simulink model "sysgenIIR_DFormI_Float"  (Simulink 7.5)
settings: Solver=VariableStepDiscrete  SolverMode=SingleTasking  StartTime=0.0  StopTime=20000  RelTol=1e-3
PreLoadFcn:
  | xlrequire('PreLoadFcn')
values from neighbouring files (symbols this model uses):
  Fs = 1 ./ block_data.params.XIncr    [sdspfscope2_r13.m]
undefined symbols (not defined in the file or in its folder): a1, a2, b0, b1, b2, One, sided
libraries: xbsIndex_r4 x59, dspobslib x6, dspstat3 x4, simulink x4, dspswit3 x2, dspsnks4 x2, xbsCopyrightNotice_r4 x1, dspsrcs4 x1
settings Model: Creator=alexc  LastModifiedBy=arvinds
settings DataIOCC: SignalLoggingName=sigsOut
settings OptimizationCC: BlockReduction=off  BooleanDataType=off  InlineInvariantSignals=on  InitFltsAndDblsToZero=on
settings DebuggingCC: SaveWithParameterizedLinksMsg=none  SignalResolutionControl=TryResolveAllWithWarning  SolverPrmCheckMsg=none  MultiTaskDSMMsg=warning  MultiTaskCondExecSysMsg=none  StrictBusMsg=None
settings HardwareCC: TargetUnknown=on
settings RTWCC: IncludeERTFirstTime=on
settings GRTTargetCC: TargetFcnLib=ansi_tfl_tmw.mat

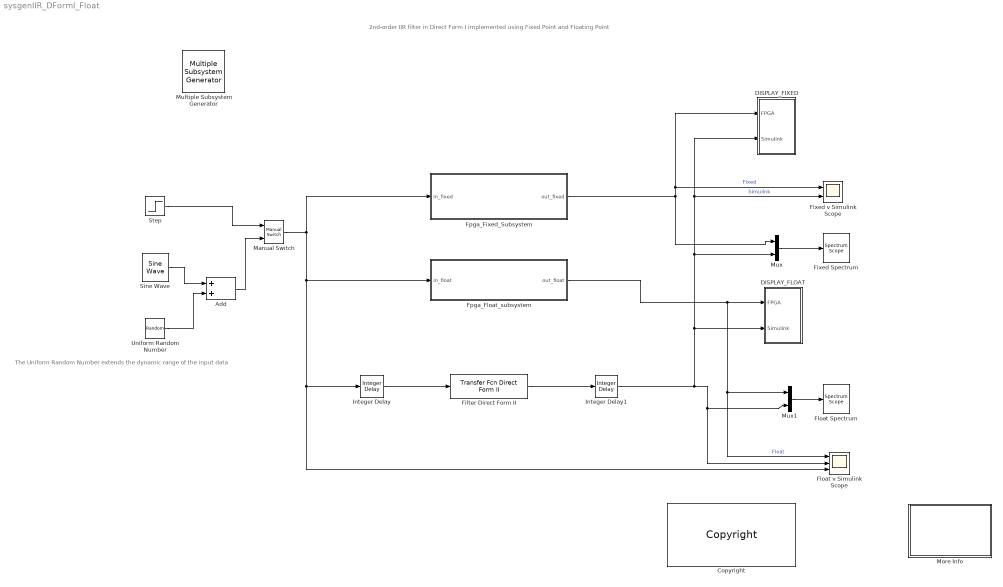
== system sysgenIIR_DFormI_Float ==
  note: 2nd-order IIR filter in Direct Form I
      | implemented using Fixed Point  and Floating Point
  note: The Uniform Random Number
      | extends the dynamic range of the input data
  Add : Sum
  Copyright : xbsCopyrightNotice_r4/Copyright  copyrighttext="Copyright (c) 2011  by  Xilinx, Inc. All rights reserved.<br><br>This file contains proprietary, confidential information of Xilinx, Inc., is distributed under license from Xilinx, Inc., and may be used, copied and/or disclosed only pursuant to the terms of a valid license agreement with Xilinx, Inc. Xilinx hereby grants you a license to use this file solely for design, simulation, implementation and creation of design files limited to Xilinx devices or technologies. Use with non-Xilinx devices or technologies is expressly prohibited and immediately terminates your license unless covered by a separate agreement.<br><br>Xilinx is providing this design, code, or information \"as-is\" solely for use in developing programs and solutions for Xilinx devices, with no obligation on the part of Xilinx to provide support. By providing this design, code, or information as one possible implementation of this feature, application or standard, Xilinx is making no representation that this implementation is free from any claims of infringement. You are responsible for obtaining any rights you may require for your implementation. Xilinx expressly disclaims any warranty whatsoever with respect to the adequacy of the implementation, including but not limited to any warranties or representations that this implementation is free from claims of infringement, implied warranties of merchantability or fitness for a particular purpose.<br><br>Xilinx products are not intended for use in life support appliances, devices, or systems. Use in such applications is expressly prohibited.<br><br>Any modifications that are made to the Source Code are done at the user's sole risk and will be unsupported.<br><br>This copyright and support notice must be retained as part of this text at all times. (c) Copyright 1995-2011 Xilinx, Inc. All rights reserved."  block_type=copyright
      settings: block_version=10.1.00
      settings: infoedit=|
      | Copyright(C) 2008 by  Xilinx, Inc. All rights reserved.<br>
      | <br>
      | This file contains proprietary, confidential information of Xilinx, Inc., is distributed under license
      | from Xilinx, Inc., and may be used, copied and/or disclosed only pursuant to the terms of a valid license
      | agreement with Xilinx, Inc. Xilinx hereby grants you a license to use this file solely for design,
      | simulation, implementation and creation of design files limited to Xilinx devices or technologies. Use
      | with non-Xilinx devices or technologies is expressly prohibited and immediately terminates your license
      | unless covered by a separate agreement.<br>
      | <br>
      | Xilinx is providing this design, code, or information "as-is" solely for use in developing programs and
      | solutions for Xilinx devices, with no obligation on the part of Xilinx to provide support. By providing
      | this design, code, or information as one possible implementation of this feature, application or standard,
      | Xilinx is making no representation that this implementation is free from any claims of infringement. You
      | are responsible for obtaining any rights you may require for your implementation. Xilinx expressly disclaims
      | any warranty whatsoever with respect to the adequacy of the implementation, including but not limited to any
      | warranties or representations that this implementation is free from claims of infringement, implied warranties
      | of merchantability or fitness for a particular purpose.<br>
      | <br>
      | Xilinx products are not intended for use in life support appliances, devices, or systems. Use in such
      | applications is expressly prohibited.<br>
      | <br>
      | Any modifications that are made to the Source Code are done at the user's sole risk and will be unsupported.<br>
      | <br>
      | This copyright and support notice must be retained as part of this text at all times.
      | (c) Copyright 1995-2008 Xilinx, Inc. All rights reserved.
  DISPLAY_FIXED : Subsystem  TreatAsAtomicUnit=on
  DISPLAY_FLOAT : Subsystem  TreatAsAtomicUnit=on
  Filter Direct Form II : simulink/Additional Math & Discrete/Additional Discrete/Transfer Fcn Direct Form II  SystemSampleTime=-1  NumCoefVec=[1 -1.6929 1]  DenCoefVec=[1.2591 0.82538]  vinit=0.0  DoSatur=off
  Fixed Spectrum : dspsnks4/Spectrum Scope  DialogController=dspdialog.SpectrumScope  DialogControllerArgs=DataTag8  SystemSampleTime=-1  ScopeProperties=off  Domain=Frequency  HorizSpan=1  UseBuffer=on  BufferSize=512  Overlap=0  inpFftLenInherit=off  FFTlength=128  numAvg=1  DisplayProperties=off  AxisGrid=on  Memory=off  FrameNumber=on  AxisLegend=on  AxisZoom=off  OpenScopeAtSimStart=on  OpenScopeImmediately=off  FigPos=[1105 390 423 236]  AxisProperties=off  XUnits=Hertz  XRange=One-sided ([0...Fs/2])  XDisplay=0  InheritXIncr=off  XIncr=1/50e6  XLabel=Samples  XLimit=Auto  YUnits=dBW/Hertz  XMax=1  XMin=0  YLabel=Magnitude, dB  LineProperties=off  LineColors=[0 1 1]|[0 0 1]|[0.1 0.6 0.1]  wintypeSpecScope=Hann  RsSpecScope=50  betaSpecScope=5  winsampSpecScope=Periodic  XAxisParamsVer=6.9
      settings: YMin=-100  YMax=0
  Fixed v Simulink Scope : Scope  NumInputPorts=2
      settings: YMin=-150~-125  YMax=150~125
  Float Spectrum : dspsnks4/Spectrum Scope  DialogController=dspdialog.SpectrumScope  DialogControllerArgs=DataTag9  SystemSampleTime=-1  ScopeProperties=off  Domain=Frequency  HorizSpan=1  UseBuffer=on  BufferSize=512  Overlap=0  inpFftLenInherit=off  FFTlength=128  numAvg=1  DisplayProperties=off  AxisGrid=on  Memory=off  FrameNumber=on  AxisLegend=on  AxisZoom=off  OpenScopeAtSimStart=on  OpenScopeImmediately=off  FigPos=[1105 390 423 236]  AxisProperties=off  XUnits=Hertz  XRange=One-sided ([0...Fs/2])  XDisplay=0  InheritXIncr=off  XIncr=1/50e6  XLabel=Samples  XLimit=Auto  YUnits=dBW/Hertz  XMax=1  XMin=0  YLabel=Magnitude, dB  LineProperties=off  LineColors=[0 1 1]|[0 0 1]|[0.1 0.6 0.1]  wintypeSpecScope=Hann  RsSpecScope=50  betaSpecScope=5  winsampSpecScope=Periodic  XAxisParamsVer=6.9
      settings: YMin=-100  YMax=0
  Float v Simulink Scope : Scope  NumInputPorts=3
      settings: YMin=-100~-100~-20  YMax=100~100~20
  Fpga_Fixed_Subsystem : Subsystem
  Fpga_Float_subsystem : Subsystem
  Integer Delay : simulink/Discrete/Integer Delay  vinit=0.0  samptime=1/Fs  NumDelays=5
  Integer Delay1 : simulink/Discrete/Integer Delay  vinit=0.0  samptime=1/Fs  NumDelays=2
  Manual Switch : simulink/Signal Routing/Manual Switch  SystemSampleTime=-1  sw=0  action=0  varsize=off
  More Info : Subsystem
      mask Display: disp('Double click\n for\n more information.')
  Multiple Subsystem Generator : xbsIndex_r4/Multiple Subsystem Generator  Tag=xlStitcher  block_type=multiple_subsystem_generator
      settings: infoedit=Multiple Subsystem\nGenerator  block_version=13.3
  Mux : Mux  Inputs=2
  Mux1 : Mux  Inputs=2
  Sine Wave : dspsrcs4/Sine Wave  Amplitude=9.99  Frequency=Fs/10  Phase=0  SampleMode=Discrete  OutComplex=Real  CompMethod=Trigonometric fcn  TableSize=Speed  SampleTime=1/Fs  SamplesPerFrame=1  dataType=double  wordLen=16  udDataType=sfix(16)  fracBitsMode=Best precision  numFracBits=14  ResetState=Restart at time zero
  Step : Step  Before=1  After=0  SampleTime=1/Fs
  Uniform Random Number : UniformRandomNumber  Minimum=-7  Maximum=7  SampleTime=1/Fs
  wires:
  Filter Direct Form II/1 -> Integer Delay1/1
  Fpga_Fixed_Subsystem/1(out_fixed) -> Mux/1, DISPLAY_FIXED/1(FPGA), Fixed v Simulink Scope/1  "Fixed"
  Step/1 -> Manual Switch/1
  Manual Switch/1 -> Fpga_Fixed_Subsystem/1(in_fixed), Fpga_Float_subsystem/1(in_float), Float v Simulink Scope/3, Integer Delay/1
  Integer Delay1/1 -> DISPLAY_FLOAT/2(Simulink), Mux/2, DISPLAY_FIXED/2(Simulink), Fixed v Simulink Scope/2, Mux1/2, Float v Simulink Scope/2  "Simulink"
  Mux/1 -> Fixed Spectrum/1
  Fpga_Float_subsystem/1(out_float) -> DISPLAY_FLOAT/1(FPGA), Mux1/1, Float v Simulink Scope/1  "Float"
  Mux1/1 -> Float Spectrum/1
  Uniform Random Number/1 -> Add/2
  Sine Wave/1 -> Add/1
  Add/1 -> Manual Switch/2
  Integer Delay/1 -> Filter Direct Form II/1

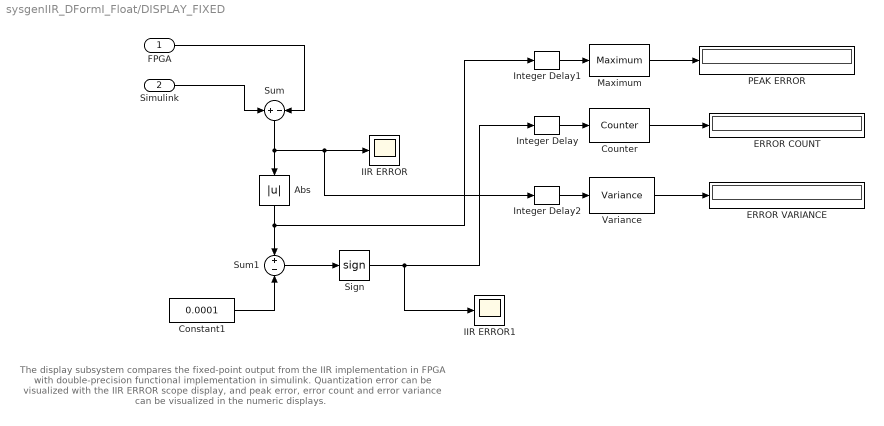
== system sysgenIIR_DFormI_Float/DISPLAY_FIXED ==
  note: The display subsystem compares the fixed-point output from the IIR implementation in FPGA
      | with double-precision functional implementation in simulink. Quantization error can be visualized
      | with the IIR ERROR scope display, and peak error, error count and error variance can be visualized
      | in the numeric displays.
  FPGA : Inport
  Simulink : Inport  Port=2
  Abs : Abs  SaturateOnIntegerOverflow=on
  Constant1 : Constant  Value=0.0001
  Counter : dspswit3/Counter  Direction=Up  CountEvent=Non-zero sample  CounterSize=User defined  MaxCount=200000000  InitialCount=0  Output=Count  HitValue=32  ResetInput=off  SamplesPerFrame=1  Ts=1  CntDtype=double  HitDtype=Logical
  ERROR COUNT : Display
  ERROR VARIANCE : Display
      settings: Format=long_e
  IIR ERROR : Scope
      settings: TimeRange=10000  YMin=-0.0006  YMax=0.0005  SaveName=ScopeData2
  IIR ERROR1 : Scope
      settings: TimeRange=10000  YMin=-0.0006  YMax=0.0005  SaveName=ScopeData3
  Integer Delay : dspobslib/Integer Delay  delay=1  ic=0  reset_popup=None
  Integer Delay1 : dspobslib/Integer Delay  delay=1  ic=0  reset_popup=None
  Integer Delay2 : dspobslib/Integer Delay  delay=1  ic=0  reset_popup=None
  Maximum : dspstat3/Maximum  DialogController=dspDDGCreate  DialogControllerArgs=DataTag1  fcn=Running  reset=None  indexBase=One  operateOver=Each column  Dimension=1  colComp=on  operation=maximum  roiEnable=off  roiType=Rectangles  roiPortion=Entire ROI  roiOutput=Individual statistics for each ROI  roiFlag=off  accumDataTypeStr=Inherit: Same as product output  accumLastDataTypeStr=Inherit: Same as product output  roundingMode=Floor  overflowMode=off
  PEAK ERROR : Display
      settings: Format=long_e
  Sign : Signum
  Sum : Sum  Inputs=+-  SaturateOnIntegerOverflow=on  InputSameDT=on  OutDataTypeStr=Inherit: Same as first input
  Sum1 : Sum  Inputs=+-  SaturateOnIntegerOverflow=on  InputSameDT=on  OutDataTypeStr=Inherit: Same as first input
  Variance : dspstat3/Variance  DialogController=dspDDGCreate  DialogControllerArgs=DataTag3  run=on  reset_popup=None  directionMode=Each column  dimension=1  treatSBRowAsCol=on  roiEnable=off  roiType=Rectangles  roiPortion=Entire ROI  roiOutput=Individual statistics for each ROI  roiFlag=off  roundingMode=Floor  overflowMode=off
  wires:
  FPGA/1 -> Sum/2
  Simulink/1 -> Sum/1
  Sum/1 -> Abs/1, IIR ERROR/1, Integer Delay2/1
  Constant1/1 -> Sum1/2
  Abs/1 -> Sum1/1, Integer Delay1/1
  Sum1/1 -> Sign/1
  Sign/1 -> Integer Delay/1, IIR ERROR1/1
  Counter/1 -> ERROR COUNT/1
  Variance/1 -> ERROR VARIANCE/1
  Maximum/1 -> PEAK ERROR/1
  Integer Delay/1 -> Counter/1
  Integer Delay1/1 -> Maximum/1
  Integer Delay2/1 -> Variance/1

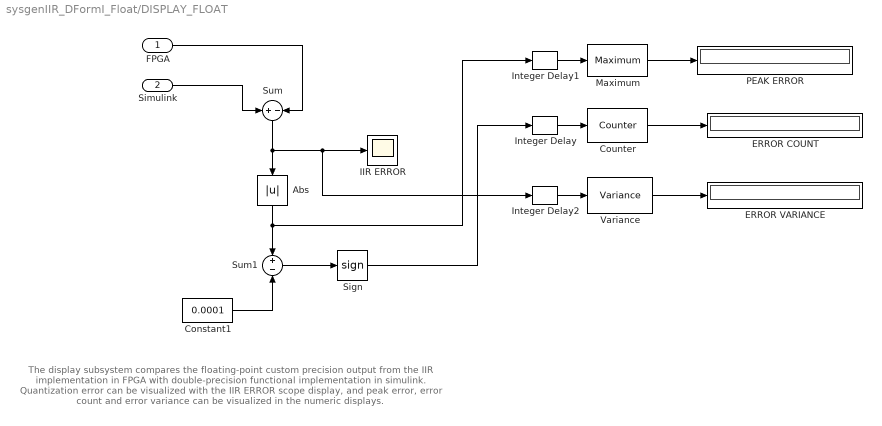
== system sysgenIIR_DFormI_Float/DISPLAY_FLOAT ==
  note: The display subsystem compares the floating-point custom precision output from the IIR implementation in FPGA
      | with double-precision functional implementation in simulink. Quantization error can be visualized
      | with the IIR ERROR scope display, and peak error, error count and error variance can be visualized
      | in the numeric displays.
  FPGA : Inport
  Simulink : Inport  Port=2
  Abs : Abs  SaturateOnIntegerOverflow=on
  Constant1 : Constant  Value=0.0001
  Counter : dspswit3/Counter  Direction=Up  CountEvent=Rising edge  CounterSize=User defined  MaxCount=200000000  InitialCount=0  Output=Count  HitValue=32  ResetInput=off  SamplesPerFrame=1  Ts=1  CntDtype=double  HitDtype=Logical
  ERROR COUNT : Display
  ERROR VARIANCE : Display
      settings: Format=long_e
  IIR ERROR : Scope
      settings: TimeRange=10000  YMin=-0.0006  YMax=0.0005  SaveName=ScopeData2
  Integer Delay : dspobslib/Integer Delay  delay=1  ic=0  reset_popup=None
  Integer Delay1 : dspobslib/Integer Delay  delay=1  ic=0  reset_popup=None
  Integer Delay2 : dspobslib/Integer Delay  delay=1  ic=0  reset_popup=None
  Maximum : dspstat3/Maximum  DialogController=dspDDGCreate  DialogControllerArgs=DataTag5  fcn=Running  reset=None  indexBase=One  operateOver=Each column  Dimension=1  colComp=on  operation=maximum  roiEnable=off  roiType=Rectangles  roiPortion=Entire ROI  roiOutput=Individual statistics for each ROI  roiFlag=off  accumDataTypeStr=Inherit: Same as product output  accumLastDataTypeStr=Inherit: Same as product output  roundingMode=Floor  overflowMode=off
  PEAK ERROR : Display
      settings: Format=long_e
  Sign : Signum
  Sum : Sum  Inputs=+-  SaturateOnIntegerOverflow=on  InputSameDT=on  OutDataTypeStr=Inherit: Same as first input
  Sum1 : Sum  Inputs=+-  SaturateOnIntegerOverflow=on  InputSameDT=on  OutDataTypeStr=Inherit: Same as first input
  Variance : dspstat3/Variance  DialogController=dspDDGCreate  DialogControllerArgs=DataTag7  run=on  reset_popup=None  directionMode=Each column  dimension=1  treatSBRowAsCol=on  roiEnable=off  roiType=Rectangles  roiPortion=Entire ROI  roiOutput=Individual statistics for each ROI  roiFlag=off  roundingMode=Floor  overflowMode=off
  wires:
  FPGA/1 -> Sum/2
  Simulink/1 -> Sum/1
  Sum/1 -> Abs/1, IIR ERROR/1, Integer Delay2/1
  Constant1/1 -> Sum1/2
  Abs/1 -> Sum1/1, Integer Delay1/1
  Sum1/1 -> Sign/1
  Sign/1 -> Integer Delay/1
  Counter/1 -> ERROR COUNT/1
  Variance/1 -> ERROR VARIANCE/1
  Maximum/1 -> PEAK ERROR/1
  Integer Delay/1 -> Counter/1
  Integer Delay1/1 -> Maximum/1
  Integer Delay2/1 -> Variance/1

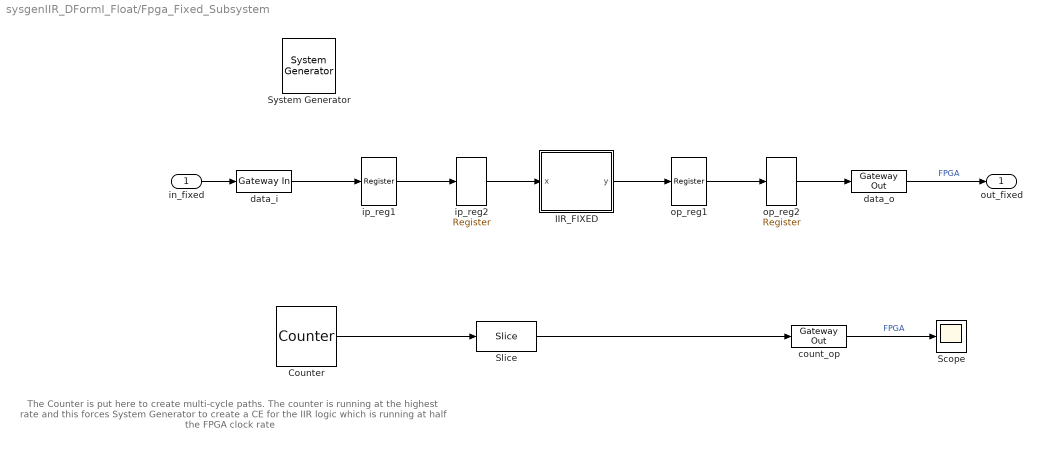
== system sysgenIIR_DFormI_Float/Fpga_Fixed_Subsystem ==
  note: The Counter is put here to create multi-cycle paths. The counter is running at the highest rate
      | and this forces System Generator  to create a CE for the IIR logic which is running at half the
      | FPGA clock rate
  in_fixed : Inport
  " System Generator" : xbsIndex_r4/ System Generator  Tag=genX  SystemSampleTime=-1  xilinxfamily=virtex6  part=xc6vlx240t  speed=-1  package=ff1156  synthesis_tool=XST  clock_wrapper=Clock Enables  directory=./fixed_timing  proj_type=Project Navigator  Synth_file=XST Defaults  Impl_file=ISE Defaults  testbench=off  simulink_period=1/(2*Fs)  sysclk_period=20  dcm_input_clock_period=100  incr_netlist=off  trim_vbits=According to Block Masks  dbl_ovrd=According to Block Masks  core_generation=According to Block Masks  run_coregen=off  deprecated_control=off  eval_field=0  block_type=sysgen
      settings: block_version=9.2.00
  Counter : xbsIndex_r4/Counter  cnt_type=Free Running  cnt_to=Inf  operation=Up  start_count=0  cnt_by_val=1  arith_type=Unsigned  n_bits=8  bin_pt=0  load_pin=off  rst=off  en=off  explicit_period=on  period=1/(2*Fs)  dbl_ovrd=off  use_behavioral_HDL=off  implementation=Fabric  block_type=counter
      settings: block_version=13.3
  IIR_FIXED : Subsystem
  Scope : Scope
      settings: SaveName=ScopeData5
  Slice : xbsIndex_r4/Slice  nbits=1  boolean_output=on  mode=Upper Bit Location + Width  bit1=0  base1=MSB of Input  bit0=0  base0=LSB of Input  dbl_ovrd=off  block_type=slice
      settings: block_version=13.3
  count_op : xbsIndex_r4/Gateway Out  hdl_port=off  timing_constraint=None  locs_specified=off  LOCs={}  block_type=gatewayout
      settings: infoedit="Gateway out block.  Converts Xilinx fixed point or floating-point type inputs into ouputs of type Simulink integer, double, or fixed point.<br><br>Hardware notes:  In hardware these blocks become top level output ports or are discarded, depending on how they are configured."  xl_area=[0 0 0 0 12 0 0]  block_version=VER_STRING_GOES_HERE
  data_i : xbsIndex_r4/Gateway In  gui_display_data_type=Fixed-point  arith_type="Signed  (2's comp)"  n_bits=data_width  bin_pt=data_binary_pt  preci_type=Single  exp_width=8  frac_width=24  quantization="Round  (unbiased: +/- Inf)"  overflow=Saturate  period=1/Fs  dbl_ovrd=off  timing_constraint=None  locs_specified=off  LOCs={}  hdl_port=on  block_type=gatewayin
      settings: infoedit="Gateway in block.  Converts inputs of type Simulink integer, double and fixed point to  Xilinx fixed point or floating-point data type.<br><br>Hardware notes:  In hardware these blocks become top level input ports."  xl_area=[0 0 0 0 12 0 0]  block_version=VER_STRING_GOES_HERE
  data_o : xbsIndex_r4/Gateway Out  hdl_port=on  timing_constraint=None  locs_specified=off  LOCs={}  block_type=gatewayout
      settings: infoedit="Gateway out block.  Converts Xilinx fixed point inputs into ouputs of type Simulink integer, double, or fixed point.<P><P>Hardware notes:  In hardware these blocks become top level output ports or are discarded, depending on how they are configured."  xl_area=[0 0 0 0 12 0 0]  block_version=VER_STRING_GOES_HERE
  ip_reg1 : xbsIndex_r4/Register  init=0  rst=off  en=off  dbl_ovrd=off  block_type=register
      settings: block_version=VER_STRING_GOES_HERE
  ip_reg2 : xbsIndex_r4/Register  init=0  rst=off  en=off  dbl_ovrd=off  block_type=register
      settings: block_version=VER_STRING_GOES_HERE
  op_reg1 : xbsIndex_r4/Register  init=0  rst=off  en=off  dbl_ovrd=off  block_type=register
      settings: block_version=VER_STRING_GOES_HERE
  op_reg2 : xbsIndex_r4/Register  init=0  rst=off  en=off  dbl_ovrd=off  block_type=register
      settings: block_version=VER_STRING_GOES_HERE
  out_fixed : Outport
  wires:
  data_i/1 -> ip_reg1/1
  ip_reg1/1 -> ip_reg2/1
  ip_reg2/1 -> IIR_FIXED/1(x)
  op_reg1/1 -> op_reg2/1
  IIR_FIXED/1(y) -> op_reg1/1
  op_reg2/1 -> data_o/1
  in_fixed/1 -> data_i/1
  data_o/1 -> out_fixed/1  "FPGA"
  count_op/1 -> Scope/1  "FPGA"
  Counter/1 -> Slice/1
  Slice/1 -> count_op/1

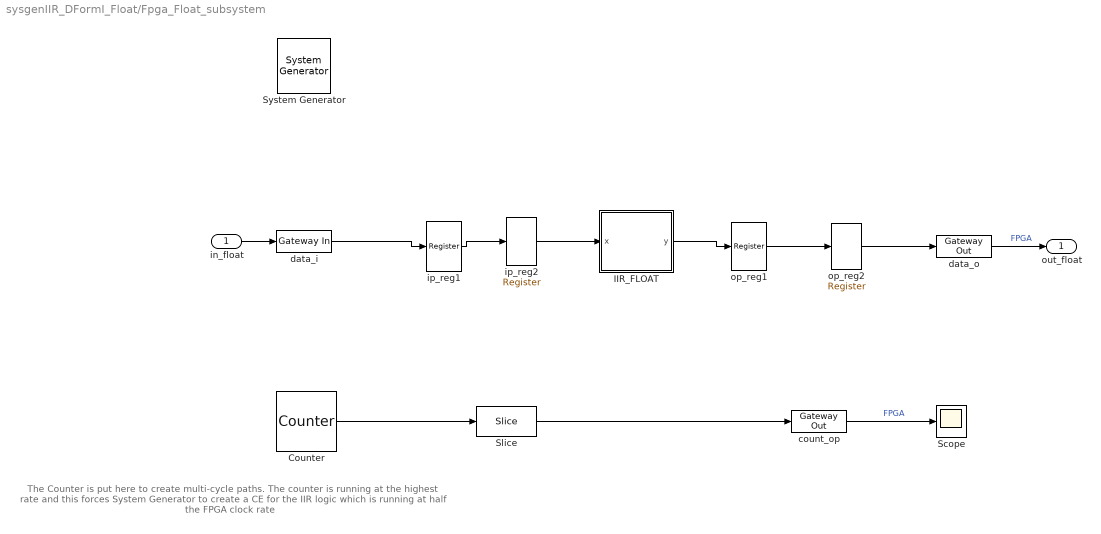
== system sysgenIIR_DFormI_Float/Fpga_Float_subsystem ==
  note: The Counter is put here to create multi-cycle paths. The counter is running at the highest rate
      | and this forces System Generator  to create a CE for the IIR logic which is running at half the
      | FPGA clock rate
  in_float : Inport
  " System Generator" : xbsIndex_r4/ System Generator  Tag=genX  SystemSampleTime=-1  xilinxfamily=virtex6  part=xc6vlx240t  speed=-1  package=ff1156  synthesis_tool=XST  clock_wrapper=Clock Enables  directory=./netlist  proj_type=Project Navigator  Synth_file=XST Defaults  Impl_file=ISE Defaults  testbench=off  simulink_period=1/(2*Fs)  sysclk_period=20  dcm_input_clock_period=100  incr_netlist=off  trim_vbits=According to Block Masks  dbl_ovrd=According to Block Masks  core_generation=According to Block Masks  run_coregen=off  deprecated_control=off  eval_field=0  block_type=sysgen
      settings: block_version=9.2.00
  Counter : xbsIndex_r4/Counter  cnt_type=Free Running  cnt_to=Inf  operation=Up  start_count=0  cnt_by_val=1  arith_type=Unsigned  n_bits=8  bin_pt=0  load_pin=off  rst=off  en=off  explicit_period=on  period=1/(2*Fs)  dbl_ovrd=off  use_behavioral_HDL=off  implementation=Fabric  block_type=counter
      settings: block_version=13.3
  IIR_FLOAT : Subsystem
  Scope : Scope
      settings: SaveName=ScopeData4
  Slice : xbsIndex_r4/Slice  nbits=1  boolean_output=on  mode=Upper Bit Location + Width  bit1=0  base1=MSB of Input  bit0=0  base0=LSB of Input  dbl_ovrd=off  block_type=slice
      settings: block_version=13.3
  count_op : xbsIndex_r4/Gateway Out  hdl_port=off  timing_constraint=None  locs_specified=off  LOCs={}  block_type=gatewayout
      settings: infoedit="Gateway out block.  Converts Xilinx fixed point or floating-point type inputs into ouputs of type Simulink integer, double, or fixed point.<br><br>Hardware notes:  In hardware these blocks become top level output ports or are discarded, depending on how they are configured."  xl_area=[0 0 0 0 12 0 0]  block_version=VER_STRING_GOES_HERE
  data_i : xbsIndex_r4/Gateway In  gui_display_data_type=Floating-point  arith_type=Floating-point  n_bits=data_width  bin_pt=data_binary_pt  preci_type=Custom  exp_width=fp_exp  frac_width=fp_frac  quantization="Round  (unbiased: +/- Inf)"  overflow=Saturate  period=1/Fs  dbl_ovrd=off  timing_constraint=None  locs_specified=off  LOCs={}  hdl_port=on  block_type=gatewayin
      settings: infoedit="Gateway in block.  Converts inputs of type Simulink integer, double and fixed point to  Xilinx fixed point or floating-point data type.<br><br>Hardware notes:  In hardware these blocks become top level input ports."  xl_area=[0 0 0 0 12 0 0]  block_version=VER_STRING_GOES_HERE
  data_o : xbsIndex_r4/Gateway Out  hdl_port=on  timing_constraint=None  locs_specified=off  LOCs={}  block_type=gatewayout
      settings: infoedit="Gateway out block.  Converts Xilinx fixed point inputs into ouputs of type Simulink integer, double, or fixed point.<P><P>Hardware notes:  In hardware these blocks become top level output ports or are discarded, depending on how they are configured."  xl_area=[0 0 0 0 12 0 0]  block_version=VER_STRING_GOES_HERE
  ip_reg1 : xbsIndex_r4/Register  init=0  rst=off  en=off  dbl_ovrd=off  block_type=register
      settings: block_version=VER_STRING_GOES_HERE
  ip_reg2 : xbsIndex_r4/Register  init=0  rst=off  en=off  dbl_ovrd=off  block_type=register
      settings: block_version=VER_STRING_GOES_HERE
  op_reg1 : xbsIndex_r4/Register  init=0  rst=off  en=off  dbl_ovrd=off  block_type=register
      settings: block_version=VER_STRING_GOES_HERE
  op_reg2 : xbsIndex_r4/Register  init=0  rst=off  en=off  dbl_ovrd=off  block_type=register
      settings: block_version=VER_STRING_GOES_HERE
  out_float : Outport
  wires:
  data_i/1 -> ip_reg1/1
  ip_reg1/1 -> ip_reg2/1
  ip_reg2/1 -> IIR_FLOAT/1(x)
  op_reg1/1 -> op_reg2/1
  IIR_FLOAT/1(y) -> op_reg1/1
  op_reg2/1 -> data_o/1
  in_float/1 -> data_i/1
  data_o/1 -> out_float/1  "FPGA"
  count_op/1 -> Scope/1  "FPGA"
  Counter/1 -> Slice/1
  Slice/1 -> count_op/1

== system sysgenIIR_DFormI_Float/More Info ==
  note: This design example shows two distinct FPGA implementations of a 2nd order IIR filter in Direct Form I,
      | and compares them to the double precision Simulink IIR filter block.
      |
      | The FPGA_FIXED_SUBSYSTEM is an IIR block 'IIIR_FIXED which is implemented with data input set to Fix32_27;
      | coefficients use 32 bit with 30 bits fractional and the adder tree usesFix32_24 notation
      |
      | The FPGA_FLOAT_SUBSYSTEM is an IIR block 'IIIR_FLOAT which is implemented using floating point block with custom
      | precision with exponent set to 7 bits and the fractional set to 20 bits
      | Therefore data and coefficients use Float_7_20
      |
      | Multiple display blocks allow the user to visualize the Power Spectrum  Density (PSD) of each
      | implementation as well as the quantization error in the DISPLAY block.
      |
      | The input is a sine wave with random noise added. if the random noise is small the fixed implementation gives good results
      | but as the dynamic range is increased the floating point implementation is better and when compared with an error window
      | the fixed implemenation is alway outside the error window.
      |
      | All the variables such as data width, coefficient width, Sample period, and coefficient values are
      | initialized in the sysgenIIR_DFormI_Float_PreLoadFcn.m file.
      |
      | A counter has been added here to create multi-cycle paths. The counter is running at the highest rate
      | and this forces System Generator  to create a CE for the IIR logic which is running at half the
      | FPGA clock rate
  note: 2nd-order IIR filter in Direct Form I
      | implemented using Fixed Point  and Floating Point

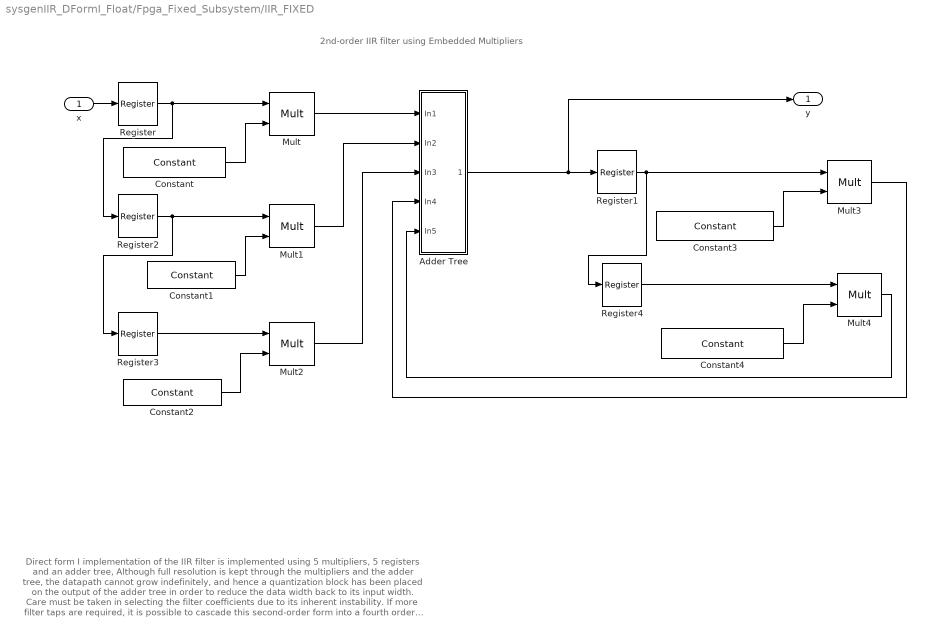
== system sysgenIIR_DFormI_Float/Fpga_Fixed_Subsystem/IIR_FIXED ==
  note: Direct form I implementation of the IIR filter is implemented using 5 multipliers, 5 registers
      | and an adder tree, Although full resolution is kept through the multipliers and the
      | adder tree, the datapath cannot grow indefinitely, and hence a quantization block has
      | been placed on the output of the adder tree in order to reduce the data width back to its
      | input width.
      | Care must be taken in selecting the filter coefficients due to its inherent instability.
      |
      | If more filter taps are required, it is possible to cascade this second-order form into a
      | fourth order cascaded filter, combine them in parallel or time share the current design
      | by saving multiple sets of coefficients in distributed memories. Similarly, the time sharing
      | approach can be used for multi-channel requirements, in which case, the coefficients can
      | be saved in distributed memories or block memories depending on the number of channels.
      |
      | Because of the feedback loop, no latency and hence no pipelining is possible in this design.
      | It is for this reason, fairly difficult to achieve high sample rate with such implementation.
  note: 2nd-order IIR filter using Embedded Multipliers
  x : Inport
  Adder Tree : Subsystem
  Constant : xbsIndex_r4/Constant  const=b0  gui_display_data_type=Fixed-point  arith_type=Signed (2's comp)  n_bits=coef_width  bin_pt=coef_binary_pt  preci_type=Single  exp_width=8  frac_width=24  explicit_period=off  period=1  equ=P=C  opselect=C  inp2=PCIN>>17  opr=+  inp1=P  carry=CIN  dbl_ovrd=off  block_type=constant
      settings: block_version=VER_STRING_GOES_HERE
  Constant1 : xbsIndex_r4/Constant  const=b1  gui_display_data_type=Fixed-point  arith_type=Signed (2's comp)  n_bits=coef_width  bin_pt=coef_binary_pt  preci_type=Single  exp_width=8  frac_width=24  explicit_period=off  period=1  equ=P=C  opselect=C  inp2=PCIN>>17  opr=+  inp1=P  carry=CIN  dbl_ovrd=off  block_type=constant
      settings: block_version=VER_STRING_GOES_HERE
  Constant2 : xbsIndex_r4/Constant  const=b2  gui_display_data_type=Fixed-point  arith_type=Signed (2's comp)  n_bits=coef_width  bin_pt=coef_binary_pt  preci_type=Single  exp_width=8  frac_width=24  explicit_period=off  period=1  equ=P=C  opselect=C  inp2=PCIN>>17  opr=+  inp1=P  carry=CIN  dbl_ovrd=off  block_type=constant
      settings: block_version=VER_STRING_GOES_HERE
  Constant3 : xbsIndex_r4/Constant  const=-a1  gui_display_data_type=Fixed-point  arith_type=Signed (2's comp)  n_bits=coef_width  bin_pt=coef_binary_pt  preci_type=Single  exp_width=8  frac_width=24  explicit_period=off  period=1  equ=P=C  opselect=C  inp2=PCIN>>17  opr=+  inp1=P  carry=CIN  dbl_ovrd=off  block_type=constant
      settings: block_version=VER_STRING_GOES_HERE
  Constant4 : xbsIndex_r4/Constant  const=-a2  gui_display_data_type=Fixed-point  arith_type=Signed (2's comp)  n_bits=coef_width  bin_pt=coef_binary_pt  preci_type=Single  exp_width=8  frac_width=24  explicit_period=off  period=1  equ=P=C  opselect=C  inp2=PCIN>>17  opr=+  inp1=P  carry=CIN  dbl_ovrd=off  block_type=constant
      settings: block_version=VER_STRING_GOES_HERE
  Mult : xbsIndex_r4/Mult  precision=User Defined  arith_type="Signed  (2's comp)"  n_bits=32  bin_pt=24  quantization="Round  (unbiased: +/- Inf)"  overflow=Saturate  en=off  latency=1  dbl_ovrd=off  use_behavioral_HDL=off  opt=Speed  use_embedded=on  optimum_pipeline=off  pipeline=off  use_rpm=off  placement_style=Rectangular shape  block_type=mult
      settings: xl_area=[0 0 0 0 0 1 0]  block_version=VER_STRING_GOES_HERE
  Mult1 : xbsIndex_r4/Mult  precision=User Defined  arith_type="Signed  (2's comp)"  n_bits=32  bin_pt=24  quantization="Round  (unbiased: +/- Inf)"  overflow=Saturate  en=off  latency=1  dbl_ovrd=off  use_behavioral_HDL=off  opt=Speed  use_embedded=on  optimum_pipeline=off  pipeline=off  use_rpm=off  placement_style=Rectangular shape  block_type=mult
      settings: xl_area=[0 0 0 0 0 1 0]  block_version=VER_STRING_GOES_HERE
  Mult2 : xbsIndex_r4/Mult  precision=User Defined  arith_type="Signed  (2's comp)"  n_bits=32  bin_pt=24  quantization="Round  (unbiased: +/- Inf)"  overflow=Saturate  en=off  latency=1  dbl_ovrd=off  use_behavioral_HDL=off  opt=Speed  use_embedded=on  optimum_pipeline=off  pipeline=off  use_rpm=off  placement_style=Rectangular shape  block_type=mult
      settings: xl_area=[0 0 0 0 0 1 0]  block_version=VER_STRING_GOES_HERE
  Mult3 : xbsIndex_r4/Mult  precision=User Defined  arith_type="Signed  (2's comp)"  n_bits=32  bin_pt=24  quantization=Truncate  overflow=Wrap  en=off  latency=0  dbl_ovrd=off  use_behavioral_HDL=off  opt=Speed  use_embedded=on  optimum_pipeline=off  pipeline=off  use_rpm=off  placement_style=Rectangular shape  block_type=mult
      settings: xl_area=[0 0 0 0 0 1 0]  block_version=VER_STRING_GOES_HERE
  Mult4 : xbsIndex_r4/Mult  precision=User Defined  arith_type="Signed  (2's comp)"  n_bits=32  bin_pt=24  quantization=Truncate  overflow=Wrap  en=off  latency=0  dbl_ovrd=off  use_behavioral_HDL=off  opt=Speed  use_embedded=on  optimum_pipeline=off  pipeline=off  use_rpm=off  placement_style=Rectangular shape  block_type=mult
      settings: xl_area=[0 0 0 0 0 1 0]  block_version=VER_STRING_GOES_HERE
  Register{,1..4} (5 alike) : xbsIndex_r4/Register  init=0  rst=off  en=off  dbl_ovrd=off  block_type=register
      settings: xl_area=[6 12 0 0 0 0 0]  block_version=VER_STRING_GOES_HERE
  y : Outport
  wires:
  x/1 -> Register/1
  Register1/1 -> Mult3/1, Register4/1
  Constant3/1 -> Mult3/2
  Mult4/1 -> Adder Tree/5(In5)
  Mult3/1 -> Adder Tree/4(In4)
  Constant4/1 -> Mult4/2
  Register4/1 -> Mult4/1
  Mult2/1 -> Adder Tree/3(In3)
  Constant2/1 -> Mult2/2
  Register3/1 -> Mult2/1
  Constant1/1 -> Mult1/2
  Register2/1 -> Register3/1, Mult1/1
  Constant/1 -> Mult/2
  Register/1 -> Register2/1, Mult/1
  Mult1/1 -> Adder Tree/2(In2)
  Mult/1 -> Adder Tree/1(In1)
  Adder Tree/1(Out1) -> y/1, Register1/1

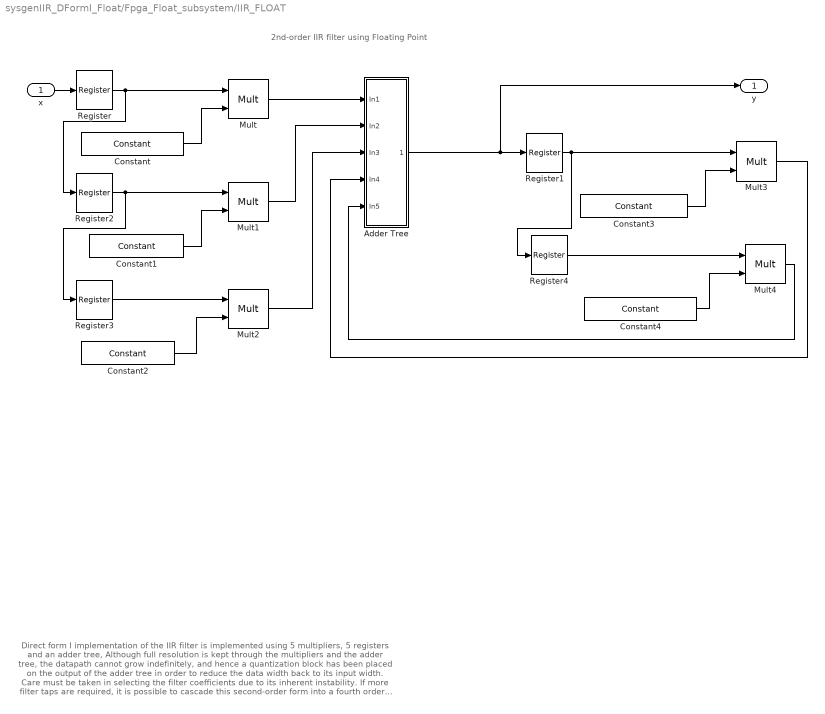
== system sysgenIIR_DFormI_Float/Fpga_Float_subsystem/IIR_FLOAT ==
  note: Direct form I implementation of the IIR filter is implemented using 5 multipliers, 5 registers
      | and an adder tree, Although full resolution is kept through the multipliers and the
      | adder tree, the datapath cannot grow indefinitely, and hence a quantization block has
      | been placed on the output of the adder tree in order to reduce the data width back to its
      | input width.
      | Care must be taken in selecting the filter coefficients due to its inherent instability.
      |
      | If more filter taps are required, it is possible to cascade this second-order form into a
      | fourth order cascaded filter, combine them in parallel or time share the current design
      | by saving multiple sets of coefficients in distributed memories. Similarly, the time sharing
      | approach can be used for multi-channel requirements, in which case, the coefficients can
      | be saved in distributed memories or block memories depending on the number of channels.
      |
      | Because of the feedback loop, no latency and hence no pipelining is possible in this design.
      | It is for this reason, fairly difficult to achieve high sample rate with such implementation and so
      | techniques like scattered.and clustered lookahead should be used
  note: 2nd-order IIR filter using Floating Point
  x : Inport
  Adder Tree : Subsystem
  Constant : xbsIndex_r4/Constant  const=b0  gui_display_data_type=Floating-point  arith_type=Floating-point  n_bits=coef_width  bin_pt=coef_binary_pt  preci_type=Custom  exp_width=fp_exp  frac_width=fp_frac  explicit_period=off  period=1  equ=P=C  opselect=C  inp2=PCIN>>17  opr=+  inp1=P  carry=CIN  dbl_ovrd=off  block_type=constant
      settings: block_version=VER_STRING_GOES_HERE
  Constant1 : xbsIndex_r4/Constant  const=b1  gui_display_data_type=Floating-point  arith_type=Floating-point  n_bits=coef_width  bin_pt=coef_binary_pt  preci_type=Custom  exp_width=fp_exp  frac_width=fp_frac  explicit_period=off  period=1  equ=P=C  opselect=C  inp2=PCIN>>17  opr=+  inp1=P  carry=CIN  dbl_ovrd=off  block_type=constant
      settings: block_version=VER_STRING_GOES_HERE
  Constant2 : xbsIndex_r4/Constant  const=b2  gui_display_data_type=Floating-point  arith_type=Floating-point  n_bits=coef_width  bin_pt=coef_binary_pt  preci_type=Custom  exp_width=fp_exp  frac_width=fp_frac  explicit_period=off  period=1  equ=P=C  opselect=C  inp2=PCIN>>17  opr=+  inp1=P  carry=CIN  dbl_ovrd=off  block_type=constant
      settings: block_version=VER_STRING_GOES_HERE
  Constant3 : xbsIndex_r4/Constant  const=-a1  gui_display_data_type=Floating-point  arith_type=Floating-point  n_bits=coef_width  bin_pt=coef_binary_pt  preci_type=Custom  exp_width=fp_exp  frac_width=fp_frac  explicit_period=off  period=1  equ=P=C  opselect=C  inp2=PCIN>>17  opr=+  inp1=P  carry=CIN  dbl_ovrd=off  block_type=constant
      settings: block_version=VER_STRING_GOES_HERE
  Constant4 : xbsIndex_r4/Constant  const=-a2  gui_display_data_type=Floating-point  arith_type=Floating-point  n_bits=coef_width  bin_pt=coef_binary_pt  preci_type=Custom  exp_width=fp_exp  frac_width=fp_frac  explicit_period=off  period=1  equ=P=C  opselect=C  inp2=PCIN>>17  opr=+  inp1=P  carry=CIN  dbl_ovrd=off  block_type=constant
      settings: block_version=VER_STRING_GOES_HERE
  Mult : xbsIndex_r4/Mult  precision=Full  arith_type="Signed  (2's comp)"  n_bits=32  bin_pt=24  quantization="Round  (unbiased: +/- Inf)"  overflow=Saturate  en=off  latency=1  dbl_ovrd=off  use_behavioral_HDL=off  opt=Speed  use_embedded=on  optimum_pipeline=off  pipeline=off  use_rpm=off  placement_style=Rectangular shape  block_type=mult
      settings: xl_area=[0 0 0 0 0 1 0]  block_version=VER_STRING_GOES_HERE
  Mult1 : xbsIndex_r4/Mult  precision=Full  arith_type="Signed  (2's comp)"  n_bits=32  bin_pt=24  quantization="Round  (unbiased: +/- Inf)"  overflow=Saturate  en=off  latency=1  dbl_ovrd=off  use_behavioral_HDL=off  opt=Speed  use_embedded=on  optimum_pipeline=off  pipeline=off  use_rpm=off  placement_style=Rectangular shape  block_type=mult
      settings: xl_area=[0 0 0 0 0 1 0]  block_version=VER_STRING_GOES_HERE
  Mult2 : xbsIndex_r4/Mult  precision=Full  arith_type="Signed  (2's comp)"  n_bits=32  bin_pt=24  quantization="Round  (unbiased: +/- Inf)"  overflow=Saturate  en=off  latency=1  dbl_ovrd=off  use_behavioral_HDL=off  opt=Speed  use_embedded=on  optimum_pipeline=off  pipeline=off  use_rpm=off  placement_style=Rectangular shape  block_type=mult
      settings: xl_area=[0 0 0 0 0 1 0]  block_version=VER_STRING_GOES_HERE
  Mult3 : xbsIndex_r4/Mult  precision=Full  arith_type="Signed  (2's comp)"  n_bits=32  bin_pt=24  quantization=Truncate  overflow=Wrap  en=off  latency=0  dbl_ovrd=off  use_behavioral_HDL=off  opt=Speed  use_embedded=on  optimum_pipeline=off  pipeline=off  use_rpm=off  placement_style=Rectangular shape  block_type=mult
      settings: xl_area=[0 0 0 0 0 1 0]  block_version=VER_STRING_GOES_HERE
  Mult4 : xbsIndex_r4/Mult  precision=Full  arith_type="Signed  (2's comp)"  n_bits=32  bin_pt=24  quantization=Truncate  overflow=Wrap  en=off  latency=0  dbl_ovrd=off  use_behavioral_HDL=off  opt=Speed  use_embedded=on  optimum_pipeline=off  pipeline=off  use_rpm=off  placement_style=Rectangular shape  block_type=mult
      settings: xl_area=[0 0 0 0 0 1 0]  block_version=VER_STRING_GOES_HERE
  Register{,1..4} (5 alike) : xbsIndex_r4/Register  init=0  rst=off  en=off  dbl_ovrd=off  block_type=register
      settings: xl_area=[6 12 0 0 0 0 0]  block_version=VER_STRING_GOES_HERE
  y : Outport
  wires:
  x/1 -> Register/1
  Register1/1 -> Mult3/1, Register4/1
  Constant3/1 -> Mult3/2
  Mult4/1 -> Adder Tree/5(In5)
  Mult3/1 -> Adder Tree/4(In4)
  Constant4/1 -> Mult4/2
  Register4/1 -> Mult4/1
  Mult2/1 -> Adder Tree/3(In3)
  Constant2/1 -> Mult2/2
  Register3/1 -> Mult2/1
  Constant1/1 -> Mult1/2
  Register2/1 -> Register3/1, Mult1/1
  Constant/1 -> Mult/2
  Register/1 -> Register2/1, Mult/1
  Mult1/1 -> Adder Tree/2(In2)
  Mult/1 -> Adder Tree/1(In1)
  Adder Tree/1(Out1) -> y/1, Register1/1

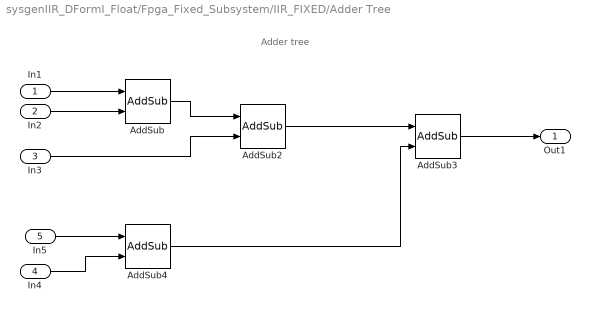
== system sysgenIIR_DFormI_Float/Fpga_Fixed_Subsystem/IIR_FIXED/Adder Tree ==
  note: Adder tree
  In1 : Inport
  In2 : Inport  Port=2
  In3 : Inport  Port=3
  In4 : Inport  Port=4
  In5 : Inport  Port=5
  AddSub : xbsIndex_r4/AddSub  mode=Addition  use_carryin=off  use_carryout=off  en=off  latency=0  precision=User Defined  arith_type="Signed  (2's comp)"  n_bits=32  bin_pt=24  quantization="Round  (unbiased: +/- Inf)"  overflow=Saturate  dbl_ovrd=off  use_behavioral_HDL=off  hw_selection=Fabric  pipelined=off  use_rpm=off  block_type=addsub
      settings: xl_area=[13 0 0 25 0 0 0]  block_version=VER_STRING_GOES_HERE
  AddSub2 : xbsIndex_r4/AddSub  mode=Addition  use_carryin=off  use_carryout=off  en=off  latency=1  precision=User Defined  arith_type="Signed  (2's comp)"  n_bits=32  bin_pt=24  quantization="Round  (unbiased: +/- Inf)"  overflow=Saturate  dbl_ovrd=off  use_behavioral_HDL=on  hw_selection=Fabric  pipelined=off  use_rpm=off  block_type=addsub
      settings: xl_area=[13 0 0 25 0 0 0]  block_version=VER_STRING_GOES_HERE
  AddSub3 : xbsIndex_r4/AddSub  mode=Addition  use_carryin=off  use_carryout=off  en=off  latency=0  precision=User Defined  arith_type="Signed  (2's comp)"  n_bits=32  bin_pt=24  quantization="Round  (unbiased: +/- Inf)"  overflow=Saturate  dbl_ovrd=off  use_behavioral_HDL=off  hw_selection=Fabric  pipelined=off  use_rpm=off  block_type=addsub
      settings: xl_area=[14 0 0 26 0 0 0]  block_version=VER_STRING_GOES_HERE
  AddSub4 : xbsIndex_r4/AddSub  mode=Addition  use_carryin=off  use_carryout=off  en=off  latency=0  precision=User Defined  arith_type="Signed  (2's comp)"  n_bits=32  bin_pt=24  quantization="Round  (unbiased: +/- Inf)"  overflow=Saturate  dbl_ovrd=off  use_behavioral_HDL=on  hw_selection=Fabric  pipelined=off  use_rpm=off  block_type=addsub
      settings: xl_area=[13 0 0 24 0 0 0]  block_version=VER_STRING_GOES_HERE
  Out1 : Outport
  wires:
  In1/1 -> AddSub/1
  In2/1 -> AddSub/2
  AddSub3/1 -> Out1/1
  In3/1 -> AddSub2/2
  AddSub/1 -> AddSub2/1
  AddSub2/1 -> AddSub3/1
  In5/1 -> AddSub4/1
  In4/1 -> AddSub4/2
  AddSub4/1 -> AddSub3/2

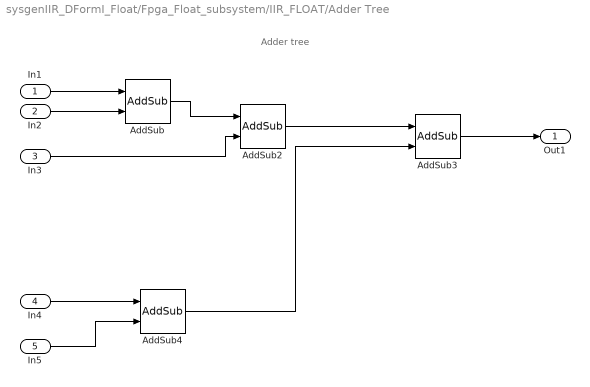
== system sysgenIIR_DFormI_Float/Fpga_Float_subsystem/IIR_FLOAT/Adder Tree ==
  note: Adder tree
  In1 : Inport
  In2 : Inport  Port=2
  In3 : Inport  Port=3
  In4 : Inport  Port=4
  In5 : Inport  Port=5
  AddSub : xbsIndex_r4/AddSub  mode=Addition  use_carryin=off  use_carryout=off  en=off  latency=0  precision=Full  arith_type="Signed  (2's comp)"  n_bits=32  bin_pt=24  quantization="Round  (unbiased: +/- Inf)"  overflow=Saturate  dbl_ovrd=off  use_behavioral_HDL=off  hw_selection=Fabric  pipelined=off  use_rpm=off  block_type=addsub
      settings: xl_area=[13 0 0 25 0 0 0]  block_version=VER_STRING_GOES_HERE
  AddSub2 : xbsIndex_r4/AddSub  mode=Addition  use_carryin=off  use_carryout=off  en=off  latency=1  precision=Full  arith_type="Signed  (2's comp)"  n_bits=32  bin_pt=24  quantization="Round  (unbiased: +/- Inf)"  overflow=Saturate  dbl_ovrd=off  use_behavioral_HDL=on  hw_selection=Fabric  pipelined=off  use_rpm=off  block_type=addsub
      settings: xl_area=[13 0 0 25 0 0 0]  block_version=VER_STRING_GOES_HERE
  AddSub3 : xbsIndex_r4/AddSub  mode=Addition  use_carryin=off  use_carryout=off  en=off  latency=0  precision=Full  arith_type="Signed  (2's comp)"  n_bits=32  bin_pt=24  quantization="Round  (unbiased: +/- Inf)"  overflow=Saturate  dbl_ovrd=off  use_behavioral_HDL=off  hw_selection=Fabric  pipelined=off  use_rpm=off  block_type=addsub
      settings: xl_area=[14 0 0 26 0 0 0]  block_version=VER_STRING_GOES_HERE
  AddSub4 : xbsIndex_r4/AddSub  mode=Addition  use_carryin=off  use_carryout=off  en=off  latency=0  precision=Full  arith_type="Signed  (2's comp)"  n_bits=32  bin_pt=24  quantization="Round  (unbiased: +/- Inf)"  overflow=Saturate  dbl_ovrd=off  use_behavioral_HDL=on  hw_selection=Fabric  pipelined=off  use_rpm=off  block_type=addsub
      settings: xl_area=[13 0 0 24 0 0 0]  block_version=VER_STRING_GOES_HERE
  Out1 : Outport
  wires:
  In1/1 -> AddSub/1
  In2/1 -> AddSub/2
  AddSub3/1 -> Out1/1
  AddSub/1 -> AddSub2/1
  AddSub2/1 -> AddSub3/1
  In4/1 -> AddSub4/1
  In5/1 -> AddSub4/2
  AddSub4/1 -> AddSub3/2
  In3/1 -> AddSub2/2
